simulink model "Simple_RC_Low_Pass_Filter"  (R2018a)
settings: Solver=VariableStepAuto  StartTime=0.0  StopTime=1  RelTol=1e-3  AbsTol=1e-3  EnableMultiTasking=on
libraries: fl_lib x7, nesl_utility x3, slctrlblks x1
settings Model: Creator=ashwin  LastModifiedBy=ashwin
settings SolverCC: AutoScaleAbsTol=off
settings DataIOCC: LimitDataPoints=on  MaxDataPoints=10000
settings OptimizationCC: LifeSpan=inf
settings DebuggingCC: AllowSymbolicDim=off  SFUnexpectedBacktrackingDiag=warning  SFNoUnconditionalDefaultTransitionDiag=warning  SFExecutionAtInitializationDiag=none
settings CodeAppCC: StateflowObjectComments=on
settings GRTTargetCC: TargetLangStandard=C89/C90 (ANSI)  GeneratePreprocessorConditionals=Disable all
settings ConfigComp: CovMetricSettings=dw  CovHtmlReporting=on  CovSaveCumulativeToWorkspaceVar=on  CovSaveSingleToWorkspaceVar=on  CovExternalEMLEnable=off  CovSFcnEnable=off
settings SimscapeCC: SimscapeLogType=all  SimscapeLogDataHistory=10000

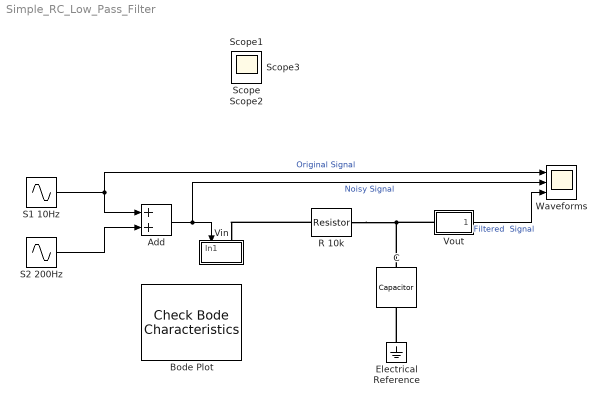
== system Simple_RC_Low_Pass_Filter ==
  Add : Sum
  Bode Plot : slctrlblks/Model Verification/Check Bode  Characteristics  InstantiateOnLoad=on  SaveOperatingPoints=off  LinearizationIOs={'/Add', 1, 'in', 'on', '';'/Vout', 1, 'out', 'on', ''}  LinearizeAt=SnapshotTimes  SnapshotTimes=[0]  TriggerType=falling  SampleTime=auto  RateConversionMethod=zoh  PreWarpFreq=10  UseExactDelayModel=off  UseFullBlockNameLabels=off  UseBusSignalLabels=off  enabled=on  stopWhenAssertionFail=off  export=off  ViewDlgPos=[233 110 510 390]  OpenViewOnLoad=off  LaunchViewOnOpen=off  FrequencyUnits=rad/s  MagnitudeUnits=dB  PhaseUnits=deg  TimeUnits=seconds  EnableUpperBound=off  UpperBoundFrequencies=[]  UpperBoundMagnitudes=[]  EnableLowerBound=off  LowerBoundFrequencies=[]  LowerBoundMagnitudes=[]
      settings: SourceProductName=Simulink Control Design
  C : fl_lib/Electrical/Electrical Elements/Capacitor  c=7.958e-7 F  r=1e-6 Ohm  g=0 1/Ohm  i_specify=off  i_priority=None  i=0 A  i_nominal_specify=off  i_nominal_unit=A  i_nominal_value=1  v_specify=off  v_priority=None  v=0 V  v_nominal_specify=off  v_nominal_unit=V  v_nominal_value=1  vc_specify=off  vc_priority=High  vc=0 V  vc_nominal_specify=off  vc_nominal_unit=V  vc_nominal_value=1
  Electrical Reference : fl_lib/Electrical/Electrical Elements/Electrical Reference
  R 10k : fl_lib/Electrical/Electrical Elements/Resistor  R=10 kOhm  i_specify=off  i_priority=None  i=0 A  i_nominal_specify=off  i_nominal_unit=A  i_nominal_value=1  v_specify=off  v_priority=None  v=0 V  v_nominal_specify=off  v_nominal_unit=V  v_nominal_value=1
  S1 10Hz : Sin  Frequency=2*pi*10  SampleTime=0
  S2 200Hz : Sin  Amplitude=0.5  Frequency=2*pi*200  SampleTime=0
  Vin : Subsystem
      mask Display: disp('Vin')
  Vout : Subsystem
      mask Display: disp('Vout')
  "Waveforms " : Scope  NumInputPorts=3
  Scope{,1..3} (4 alike) : Scope
  wires:
  S2 200Hz/1 -> Add/2
  S1 10Hz/1 -> "Waveforms "/1, Add/1  "Original Signal"
  Add/1 -> Vin/1(In1), "Waveforms "/2  "Noisy Signal"
  Vout/1(Out1) -> "Waveforms "/3  "Filtered  Signal"
  connections:
  Vout/LConn1 -- C/LConn1 -- R 10k/RConn1
  Electrical Reference/LConn1 -- C/RConn1
  R 10k/LConn1 -- Vin/LConn1

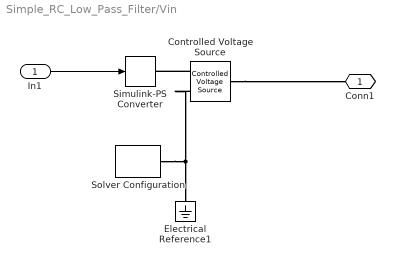
== system Simple_RC_Low_Pass_Filter/Vin ==
  In1 : Inport
  Controlled Voltage Source : fl_lib/Electrical/Electrical Sources/Controlled Voltage Source
  Electrical Reference1 : fl_lib/Electrical/Electrical Elements/Electrical Reference
  Simulink-PS Converter : nesl_utility/Simulink-PS Converter  PhysicalDomain=network_engine_domain  SubClassName=ps_input  LeftPortType=input  RightPortType=output  PseudoPeriodic=off  Frequencies=[]  NoiseDistribution=none  NoiseParameters=[]  Unit=1  AffineConversion=off  FilteringAndDerivatives=zero  SimscapeFilterOrder=1  InputFilterTimeConstant=0.001  UdotUserProvided=1
  Solver Configuration : nesl_utility/Solver Configuration  PhysicalDomain=network_engine_domain  SubClassName=solver  LeftPortType=input  RightPortType=generic  Tones=[]  Harmonics=[]  SimulateNoise=off  Profile=off  UseLocalSampling=off  EnableSwitchedLinearOptims=on  FrequencyDomain=off  UseCCode=off  RelTol=0.001  AbsTol=1e-06  MinStep=1e-09  ToWorkspace=off  RevertToSquareIcSolve=off  NumHomotopyIterations=100  PhasorMode=off  PhasorModeNumHarmonics=1  DoDC=off  ResidualTolerance=1e-09  UseLocalSolver=off  LocalSolverChoice=NE_BACKWARD_EULER_ADVANCER  LocalSolverSampleTime=0.001  DoFixedCost=off  MaxNonlinIter=3  MaxModeIter=2  LinearAlgebra=Sparse  EquationFormulation=NE_TIME_EF  DelaysMemoryBudget=1024  AutomaticFiltering=on  FilteringTimeConstant=0.001
  Conn1 : PMIOPort  Side=Left
  wires:
  In1/1 -> Simulink-PS Converter/1
  connections:
  Controlled Voltage Source/RConn2 -- Solver Configuration/RConn1 -- Electrical Reference1/LConn1
  Controlled Voltage Source/LConn1 -- Conn1/RConn1
  Controlled Voltage Source/RConn1 -- Simulink-PS Converter/RConn1

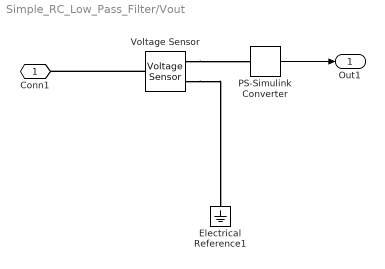
== system Simple_RC_Low_Pass_Filter/Vout ==
  Electrical Reference1 : fl_lib/Electrical/Electrical Elements/Electrical Reference
  PS-Simulink Converter : nesl_utility/PS-Simulink Converter  PhysicalDomain=network_engine_domain  SubClassName=ps_output  LeftPortType=input  RightPortType=output  PseudoPeriodic=off  Frequencies=[]  Unit=1  AffineConversion=off
  Voltage Sensor : fl_lib/Electrical/Electrical Sensors/Voltage Sensor
  Conn1 : PMIOPort  Side=Left
  Out1 : Outport
  wires:
  PS-Simulink Converter/1 -> Out1/1
  connections:
  Voltage Sensor/RConn2 -- Electrical Reference1/LConn1
  Voltage Sensor/LConn1 -- Conn1/RConn1
  Voltage Sensor/RConn1 -- PS-Simulink Converter/LConn1
